simulink model "buck"  (R2024b)
settings: Solver=ode23tb  StartTime=0.0  StopTime=0.05  MaxStep=1e-6  RelTol=1e-5  AbsTol=1e-7
PostLoadFcn:
  | p=fileparts(get_param(bdroot,'FileName')); Simulink.fileGenControl('set','CacheFolder',fullfile(p,'archive','cache'),'CodeGenFolder',fullfile(p,'archive','codegen'),'createDir',true);
libraries: spsParallelRLCBranchLib x3, spsCurrentMeasurementLib x1, spsDCVoltageSourceLib x1, spsDiodeLib x1, spsMosfetLib x1, spsVoltageMeasurementLib x1, sps_lib x1
settings Model: Creator=zzf  LastModifiedBy=zzf
settings HardwareCC: ProdBitPerPointer=32  ProdBitPerSizeT=32  ProdBitPerPtrDiffT=32  ProdWordSize=32  ProdHWDeviceType=Intel->x86-32 (Windows32)
settings SFSimCC: SimCustomHeaderCode="#include \"pid.h\""  SimCustomInitializer=pid_reset(); pid_set_tunings(0.01,10.0,1e-6); pid_set_limits(0.0,0.95); pid_set_dfilter(0.0002); pid_set_overcurrent(-1.0,0.0);  SimUserSources=pid.cpp  SimUserIncludeDirs=D:\buck_simulink  SimTargetLang=C++

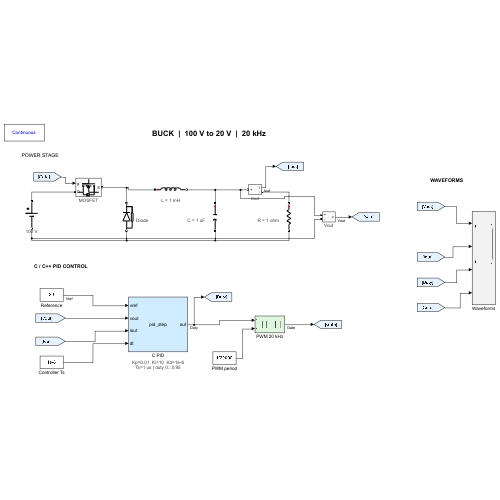
[thumbnail: Simulink's stored preview of the top-level diagram]
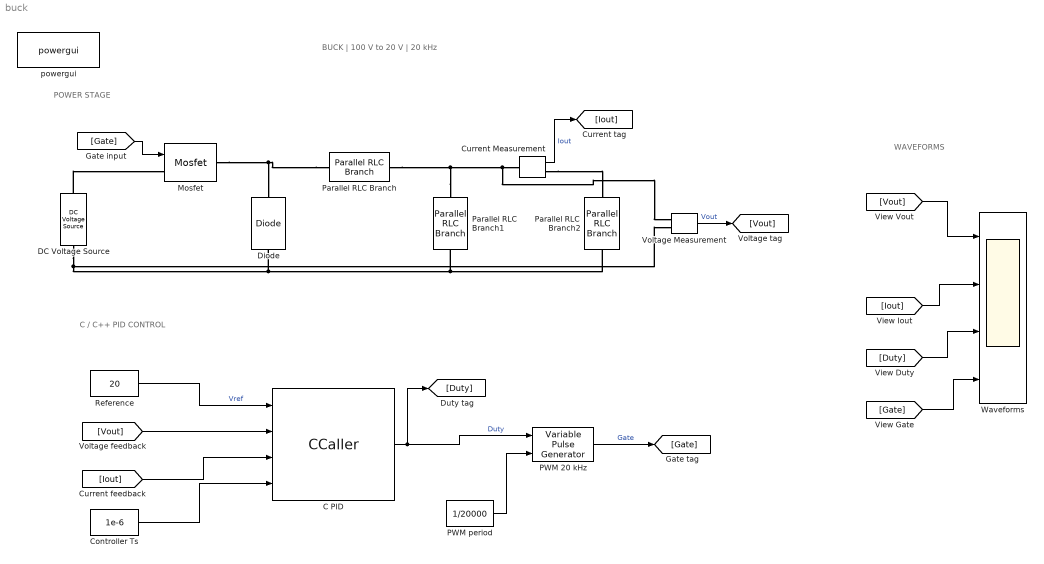
== system buck ==
  note: BUCK | 100 V to 20 V | 20 kHz
  note: POWER STAGE
  note: C / C++ PID CONTROL
  note: WAVEFORMS
  C PID : CCaller  FunctionName=pid_step  PortSpecificationStruct="%)30     .    F @   8    (     @         %    \"     4    !     0         %  0 \"0    $    _    07)G3F%M90  4&]R=$YA;64 4V-O<&4     26YD97@     5'EP90      4VEZ90      27-';&]B86P   X    P    !@    @    $          4    (     0    ,    !         !   P!O=70 #@   #     &    \"     0         !0    @    !     P    $         $  # &]U=  .    .     8    (    !          %    \"     $    &     0         0   ...(+2583 chars)"  SampleTime=1e-6
      settings: AttributesFormatString="Kp=0.01  Ki=10  Kd=1e-6\\nTs=1 us | duty 0...0.95"
  Controller Ts : Constant  Value=1e-6
  Current Measurement : spsCurrentMeasurementLib/Current Measurement  PhasorSimulation=off  OutputType=Complex  PSBequivalent=0
      settings: AttributesFormatString=Iout
  DC Voltage Source : spsDCVoltageSourceLib/DC Voltage Source  Amplitude=100  Measurements=None
      settings: AttributesFormatString=100 V
  Diode : spsDiodeLib/Diode  Ron=0.001  Lon=0  Vf=0.8  IC=0  UseSnubber=0  Rs=500  Cs=250e-9  Measurements=off
      settings: AttributesFormatString=Diode
  Mosfet : spsMosfetLib/Mosfet  Ron=0.1  Lon=0  Rd=0.01  Vfd=0  IC=0  Rs=1e5  Cs=inf  Measurements=off
      settings: AttributesFormatString=MOSFET
  PWM 20 kHz : VariablePulseGenerator  SampleTime=1e-6
  PWM period : Constant  Value=1/20000
  Parallel RLC Branch : spsParallelRLCBranchLib/Parallel RLC Branch  LConnTagsString=a  RConnTagsString=__new0  BranchType=L  Resistance=1  Inductance=1e-3  SetiL0=off  InitialCurrent=0  Capacitance=1e-6  Setx0=off  InitialVoltage=0  Measurements=None
      settings: AttributesFormatString=L = 1 mH
  Parallel RLC Branch1 : spsParallelRLCBranchLib/Parallel RLC Branch  LConnTagsString=a  RConnTagsString=__new0  BranchType=C  Resistance=1  Inductance=1e-3  SetiL0=off  InitialCurrent=0  Capacitance=1e-6  Setx0=off  InitialVoltage=0  Measurements=None
      settings: AttributesFormatString=C = 1 uF
  Parallel RLC Branch2 : spsParallelRLCBranchLib/Parallel RLC Branch  LConnTagsString=a  RConnTagsString=__new0  BranchType=R  Resistance=10  Inductance=1e-3  SetiL0=off  InitialCurrent=0  Capacitance=1e-6  Setx0=off  InitialVoltage=0  Measurements=None
      settings: AttributesFormatString=R = 1 ohm
  Reference : Constant  Value=20
  Voltage Measurement : spsVoltageMeasurementLib/Voltage Measurement  PhasorSimulation=off  OutputType=Complex  PSBequivalent=0
      settings: AttributesFormatString=Vout
  Waveforms : Scope  NumInputPorts=4
  powergui : sps_lib/powergui  Priority=1  SimulationMode=Continuous  SampleTime=50e-6  frequency=60  Iterations=50  frequencyindice=0  Pbase=100e6  ErrMax=1e-4  UnitsV=kV  UnitsW=MW  buscounter=0  FunctionMessages=off  echomessages=off  EnableUseOfTLC=off  CurrentSourceSwitches=off  DisableSnubberDevices=off  DisableRonSwitches=off  DisableVfSwitches=off  DisplayEquations=off  AutomaticDiscreteSolvers=off  SolverType=Tustin/Backward Euler (TBE)  Interpol=off  ExternalGateDelay=off  methode=off  Ts=100  x0status=blocks  SPID=on  SwTol=0  HookPort=off  NonlinearTolerance=1e-4  nMaxIteration=100  ContinueOnMaxIteration=off  RestoreLinks=warning  ResistiveCurrentMeasurement=off  Frange=[0:2:500]  Ylog=off  Xlog=on  ShowGrid=off  save=off  variable=ZData  structure=0  ZoomFFT=off  StartTime=0.0  cycles=1  DisplayStyle=1  fundamental=60  FreqAxis=off  MaxFrequency=1000  frequencyindicesteady=1  RmsSteady=1  display=off
  wires:
  Reference/1 -> C PID/1  "Vref"
  [Vout] -> C PID/2
  [Iout] -> C PID/3
  Controller Ts/1 -> C PID/4
  C PID/1 -> PWM 20 kHz/1, [Duty]  "Duty"
  PWM period/1 -> PWM 20 kHz/2
  PWM 20 kHz/1 -> [Gate]  "Gate"
  Voltage Measurement/1 -> [Vout]  "Vout"
  Current Measurement/1 -> [Iout]  "Iout"
  [Vout] -> Waveforms/1
  [Iout] -> Waveforms/2
  [Duty] -> Waveforms/3
  [Gate] -> Waveforms/4
  [Gate] -> Mosfet/1
  connections:
  DC Voltage Source/RConn1 -- Mosfet/LConn1
  Parallel RLC Branch/LConn1 -- Mosfet/RConn1 -- Diode/RConn1
  Parallel RLC Branch1/LConn1 -- Parallel RLC Branch/RConn1 -- Current Measurement/LConn1 -- Voltage Measurement/LConn1
  Current Measurement/RConn1 -- Parallel RLC Branch2/LConn1
  Diode/LConn1 -- DC Voltage Source/LConn1 -- Voltage Measurement/LConn2 -- Parallel RLC Branch1/RConn1 -- Parallel RLC Branch2/RConn1
